simulink model "N_scheme_RS"  (R2024b)
settings: Solver=VariableStepAuto  StartTime=0.0  StopTime=10.0  RelTol=1e-3
values from neighbouring files (symbols this model uses):
  a_n = (a_max + a_min)/2    (= 126)    [p14.m]
  b_n = (b_max + b_min)/2    (= 40)    [p14.m]
  c_n = (c_max + c_min)/2    (= 0.1)    [p14.m]
  Ga = 0.01    [p14.m]
  Gf = 1/(Kd*Gs)    (= 0.166666666667)    [p14.m]
  Gs = 1    [p14.m]
  Wa = (a_max - a_min)/2    (= 22)    [p14.m]
  Wb = (b_max - b_min)/2    (= 12)    [p14.m]
  Wc = (c_max - c_min)/2    (= 0.015)    [p14.m]
libraries: cstblocks x1
settings Model: Creator=adrian  LastModifiedBy=adrian

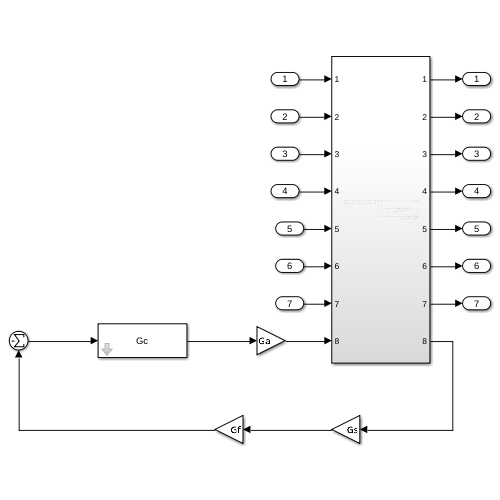
[thumbnail: Simulink's stored preview of the top-level diagram]
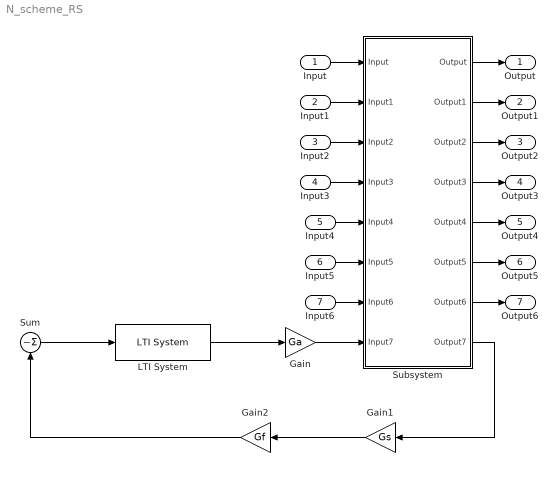
== system N_scheme_RS ==
  Input : Inport
  Input1 : Inport  Port=2
  Input2 : Inport  Port=3
  Input3 : Inport  Port=4
  Input4 : Inport  Port=5
  Input5 : Inport  Port=6
  Input6 : Inport  Port=7
  Gain : Gain  Gain=Ga
  Gain1 : Gain  Gain=Gs
  Gain2 : Gain  Gain=Gf
  LTI System : cstblocks/LTI System  sys=Gc  IC=[]  PadeOrder=0
  Subsystem : Subsystem
  Sum : Sum  Inputs=|-
  Output : Outport
  Output1 : Outport  Port=2
  Output2 : Outport  Port=3
  Output3 : Outport  Port=4
  Output4 : Outport  Port=5
  Output5 : Outport  Port=6
  Output6 : Outport  Port=7
  wires:
  LTI System/1 -> Gain/1
  Gain1/1 -> Gain2/1
  Sum/1 -> LTI System/1
  Gain/1 -> Subsystem/8(Input7)
  Subsystem/8(Output7) -> Gain1/1
  Input/1 -> Subsystem/1(Input)
  Input1/1 -> Subsystem/2(Input1)
  Input3/1 -> Subsystem/4(Input3)
  Input2/1 -> Subsystem/3(Input2)
  Input6/1 -> Subsystem/7(Input6)
  Input5/1 -> Subsystem/6(Input5)
  Input4/1 -> Subsystem/5(Input4)
  Subsystem/1(Output) -> Output/1
  Subsystem/2(Output1) -> Output1/1
  Subsystem/4(Output3) -> Output3/1
  Subsystem/3(Output2) -> Output2/1
  Subsystem/7(Output6) -> Output6/1
  Subsystem/6(Output5) -> Output5/1
  Subsystem/5(Output4) -> Output4/1
  Gain2/1 -> Sum/1

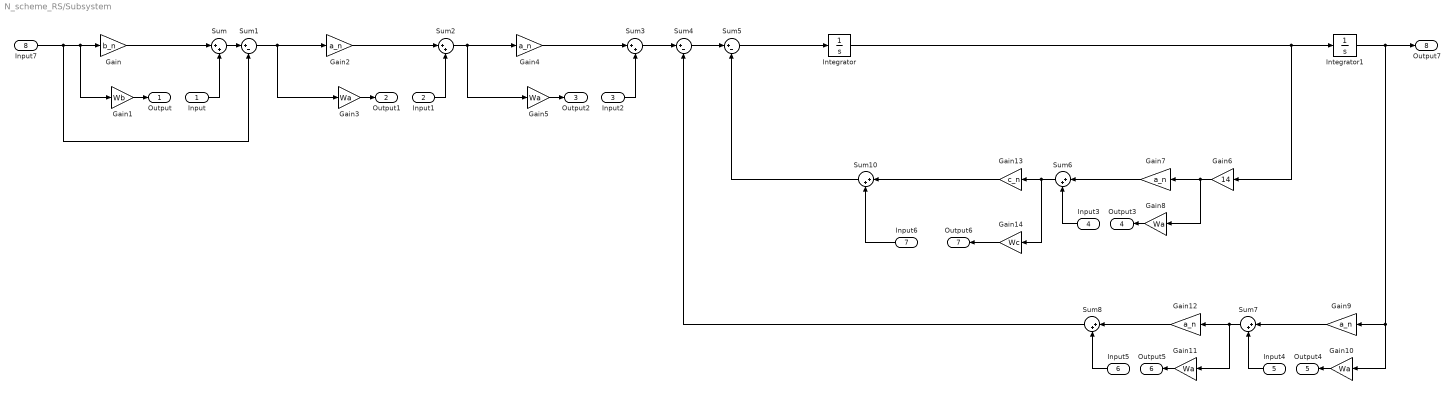
== system N_scheme_RS/Subsystem ==
  Input : Inport
  Input1 : Inport  Port=2
  Input2 : Inport  Port=3
  Input3 : Inport  Port=4
  Input4 : Inport  Port=5
  Input5 : Inport  Port=6
  Input6 : Inport  Port=7
  Input7 : Inport  Port=8
  Gain : Gain  Gain=b_n
  Gain1 : Gain  Gain=Wb
  Gain{3,5,8,10..11} (5 alike) : Gain  Gain=Wa
  Gain{2,4,7,9,12} (5 alike) : Gain  Gain=a_n
  Gain13 : Gain  Gain=c_n
  Gain14 : Gain  Gain=Wc
  Gain6 : Gain  Gain=14
  Integrator : Integrator
  Integrator1 : Integrator
  Sum{,2..3,6..8,10} (7 alike) : Sum  Inputs=|++
  Sum1 : Sum  Inputs=|+-
  Sum4 : Sum  Inputs=|+-
  Sum5 : Sum  Inputs=|+-
  Output : Outport
  Output1 : Outport  Port=2
  Output2 : Outport  Port=3
  Output3 : Outport  Port=4
  Output4 : Outport  Port=5
  Output5 : Outport  Port=6
  Output6 : Outport  Port=7
  Output7 : Outport  Port=8
  wires:
  Input7/1 -> Sum1/2, Gain/1, Gain1/1
  Gain1/1 -> Output/1
  Gain/1 -> Sum/1
  Input/1 -> Sum/2
  Sum/1 -> Sum1/1
  Input1/1 -> Sum2/2
  Gain2/1 -> Sum2/1
  Gain3/1 -> Output1/1
  Sum1/1 -> Gain3/1, Gain2/1
  Sum2/1 -> Gain4/1, Gain5/1
  Gain5/1 -> Output2/1
  Gain4/1 -> Sum3/1
  Input2/1 -> Sum3/2
  Sum4/1 -> Sum5/1
  Sum5/1 -> Integrator/1
  Sum3/1 -> Sum4/1
  Integrator/1 -> Gain6/1, Integrator1/1
  Gain6/1 -> Gain8/1, Gain7/1
  Gain8/1 -> Output3/1
  Gain7/1 -> Sum6/1
  Input3/1 -> Sum6/2
  Input4/1 -> Sum7/2
  Gain9/1 -> Sum7/1
  Gain10/1 -> Output4/1
  Integrator1/1 -> Output7/1, Gain9/1, Gain10/1
  Sum7/1 -> Gain11/1, Gain12/1
  Gain11/1 -> Output5/1
  Gain12/1 -> Sum8/1
  Input5/1 -> Sum8/2
  Sum8/1 -> Sum4/2
  Sum6/1 -> Gain14/1, Gain13/1
  Gain14/1 -> Output6/1
  Gain13/1 -> Sum10/1
  Input6/1 -> Sum10/2
  Sum10/1 -> Sum5/2
